simulink model "Normal_Multiplier"  (R2021a)
settings: Solver=FixedStepAuto  StartTime=0.0  StopTime=322.56  FixedStep=0.01  RelTol=1e-3
(part 1 of 3)
settings Model: SimulationMode=rapid-accelerator  Creator=PC  LastModifiedBy=PC
settings DataIOCC: ExternalInput=[u]
settings HardwareCC: ProdHWDeviceType=AMD->x86-64 (Windows64)

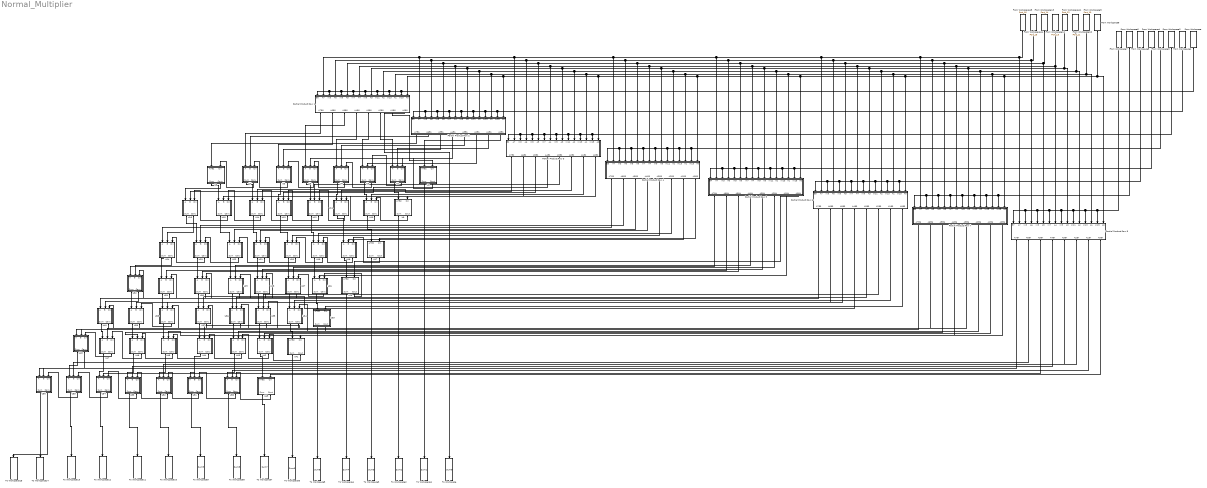
== system Normal_Multiplier ==
  From Workspace : FromWorkspace  VariableName=Port_1
  From Workspace1 : FromWorkspace  VariableName=Port_2
  From Workspace10 : FromWorkspace  VariableName=Port_11
  From Workspace11 : FromWorkspace  VariableName=Port_12
  From Workspace12 : FromWorkspace  VariableName=Port_13
  From Workspace13 : FromWorkspace  VariableName=Port_14
  From Workspace14 : FromWorkspace  VariableName=Port_15
  From Workspace15 : FromWorkspace  VariableName=Port_16
  From Workspace2 : FromWorkspace  VariableName=Port_3
  From Workspace3 : FromWorkspace  VariableName=Port_4
  From Workspace4 : FromWorkspace  VariableName=Port_5
  From Workspace5 : FromWorkspace  VariableName=Port_6
  From Workspace6 : FromWorkspace  VariableName=Port_7
  From Workspace7 : FromWorkspace  VariableName=Port_8
  From Workspace8 : FromWorkspace  VariableName=Port_9
  From Workspace9 : FromWorkspace  VariableName=Port_10
  Partial Product Row 1 : Subsystem
  Partial Product Row 2 : Subsystem
  Partial Product Row 3 : Subsystem
  Partial Product Row 4 : Subsystem
  Partial Product Row 5 : Subsystem
  Partial Product Row 6 : Subsystem
  Partial Product Row 7 : Subsystem
  Partial Product Row 8 : Subsystem
  To Workspace : ToWorkspace  VariableName=Sum0  SampleTime=0.01
      settings: Save2DSignal=2-D array (concatenate along first dimension)
  To Workspace1 : ToWorkspace  VariableName=Sum1  SampleTime=0.01
      settings: Save2DSignal=2-D array (concatenate along first dimension)
  To Workspace10 : ToWorkspace  VariableName=Sum10  SampleTime=0.01
      settings: Save2DSignal=2-D array (concatenate along first dimension)
  To Workspace11 : ToWorkspace  VariableName=Sum11  SampleTime=0.01
      settings: Save2DSignal=2-D array (concatenate along first dimension)
  To Workspace12 : ToWorkspace  VariableName=Sum12  SampleTime=0.01
      settings: Save2DSignal=2-D array (concatenate along first dimension)
  To Workspace13 : ToWorkspace  VariableName=Sum13  SampleTime=0.01
      settings: Save2DSignal=2-D array (concatenate along first dimension)
  To Workspace14 : ToWorkspace  VariableName=Sum14  SampleTime=0.01
      settings: Save2DSignal=2-D array (concatenate along first dimension)
  To Workspace15 : ToWorkspace  VariableName=Sum15  SampleTime=0.01
      settings: Save2DSignal=2-D array (concatenate along first dimension)
  To Workspace2 : ToWorkspace  VariableName=Sum2  SampleTime=0.01
      settings: Save2DSignal=2-D array (concatenate along first dimension)
  To Workspace3 : ToWorkspace  VariableName=Sum3  SampleTime=0.01
      settings: Save2DSignal=2-D array (concatenate along first dimension)
  To Workspace4 : ToWorkspace  VariableName=Sum4  SampleTime=0.01
      settings: Save2DSignal=2-D array (concatenate along first dimension)
  To Workspace5 : ToWorkspace  VariableName=Sum5  SampleTime=0.01
      settings: Save2DSignal=2-D array (concatenate along first dimension)
  To Workspace6 : ToWorkspace  VariableName=Sum6  SampleTime=0.01
      settings: Save2DSignal=2-D array (concatenate along first dimension)
  To Workspace7 : ToWorkspace  VariableName=Sum7  SampleTime=0.01
      settings: Save2DSignal=2-D array (concatenate along first dimension)
  To Workspace8 : ToWorkspace  VariableName=Sum8  SampleTime=0.01
      settings: Save2DSignal=2-D array (concatenate along first dimension)
  To Workspace9 : ToWorkspace  VariableName=Sum9  SampleTime=0.01
      settings: Save2DSignal=2-D array (concatenate along first dimension)
  U1 : Subsystem
  U10 : Subsystem
  U11 : Subsystem
  U12 : Subsystem
  U13 : Subsystem
  U14 : Subsystem
  U15 : Subsystem
  U16 : Subsystem
  U17 : Subsystem
  U18 : Subsystem
  U19 : Subsystem
  U2 : Subsystem
  U20 : Subsystem
  U21 : Subsystem
  U22 : Subsystem
  U23 : Subsystem
  U24 : Subsystem
  U25 : Subsystem
  U26 : Subsystem
  U27 : Subsystem
  U28 : Subsystem
  U29 : Subsystem
  U3 : Subsystem
  U30 : Subsystem
  U31 : Subsystem
  U32 : Subsystem
  U33 : Subsystem
  U34 : Subsystem
  U35 : Subsystem
  U36 : Subsystem
  U37 : Subsystem
  U38 : Subsystem
  U39 : Subsystem
  U4 : Subsystem
  U40 : Subsystem
  U41 : Subsystem
  U42 : Subsystem
  U43 : Subsystem
  U44 : Subsystem
  U45 : Subsystem
  U46 : Subsystem
  U47 : Subsystem
  U48 : Subsystem
  U49 : Subsystem
  U5 : Subsystem
  U50 : Subsystem
  U51 : Subsystem
  U52 : Subsystem
  U53 : Subsystem
  U54 : Subsystem
  U55 : Subsystem
  U56 : Subsystem
  U6 : Subsystem
  U7 : Subsystem
  U8 : Subsystem
  U9 : Subsystem
  wires:
  From Workspace8/1 -> Partial Product Row 8/16(A0), Partial Product Row 7/16(A0), Partial Product Row 6/16(A0), Partial Product Row 4/16(A0), Partial Product Row 3/16(A0), Partial Product Row 1/16(A0), Partial Product Row 2/16(A0), Partial Product Row 5/16(A0)
  From Workspace9/1 -> Partial Product Row 8/14(A1), Partial Product Row 7/14(A1), Partial Product Row 4/14(A1), Partial Product Row 1/14(A1), Partial Product Row 2/14(A1), Partial Product Row 3/14(A1), Partial Product Row 5/14(A1), Partial Product Row 6/14(A1)
  From Workspace10/1 -> Partial Product Row 8/12(A2), Partial Product Row 7/12(A2), Partial Product Row 5/12(A2), Partial Product Row 4/12(A2), Partial Product Row 3/12(A2), Partial Product Row 1/12(A2), Partial Product Row 2/12(A2), Partial Product Row 6/12(A2)
  From Workspace11/1 -> Partial Product Row 8/10(A3), Partial Product Row 6/10(A3), Partial Product Row 4/10(A3), Partial Product Row 3/10(A3), Partial Product Row 1/10(A3), Partial Product Row 2/10(A3), Partial Product Row 5/10(A3), Partial Product Row 7/10(A3)
  From Workspace12/1 -> Partial Product Row 8/8(A4), Partial Product Row 6/8(A4), Partial Product Row 4/8(A4), Partial Product Row 3/8(A4), Partial Product Row 1/8(A4), Partial Product Row 2/8(A4), Partial Product Row 5/8(A4), Partial Product Row 7/8(A4)
  From Workspace13/1 -> Partial Product Row 8/6(A5), Partial Product Row 6/6(A5), Partial Product Row 4/6(A5), Partial Product Row 3/6(A5), Partial Product Row 1/6(A5), Partial Product Row 2/6(A5), Partial Product Row 5/6(A5), Partial Product Row 7/6(A5)
  From Workspace14/1 -> Partial Product Row 8/4(A6), Partial Product Row 7/4(A6), Partial Product Row 6/4(A6), Partial Product Row 5/4(A6), Partial Product Row 4/4(A6), Partial Product Row 3/4(A6), Partial Product Row 1/4(A6), Partial Product Row 2/4(A6)
  From Workspace15/1 -> Partial Product Row 7/2(A7), Partial Product Row 5/2(A7), Partial Product Row 4/2(A7), Partial Product Row 3/2(A7), Partial Product Row 1/2(A7), Partial Product Row 2/2(A7), Partial Product Row 6/2(A7), Partial Product Row 8/2(A7)
  From Workspace/1 -> Partial Product Row 1/3(In3), Partial Product Row 1/1(B0), Partial Product Row 1/5(In5), Partial Product Row 1/7(In7), Partial Product Row 1/9(In9), Partial Product Row 1/11(In11), Partial Product Row 1/13(In13), Partial Product Row 1/15(In15)
  From Workspace1/1 -> Partial Product Row 2/15(In15), Partial Product Row 2/5(In5), Partial Product Row 2/3(In3), Partial Product Row 2/1(B1), Partial Product Row 2/7(In7), Partial Product Row 2/9(In9), Partial Product Row 2/11(In11), Partial Product Row 2/13(In13)
  From Workspace2/1 -> Partial Product Row 3/13(In13), Partial Product Row 3/7(In7), Partial Product Row 3/5(In5), Partial Product Row 3/3(In3), Partial Product Row 3/1(B2), Partial Product Row 3/9(In9), Partial Product Row 3/11(In11), Partial Product Row 3/15(In15)
  From Workspace3/1 -> Partial Product Row 4/15(In15), Partial Product Row 4/13(In13), Partial Product Row 4/11(In11), Partial Product Row 4/9(In9), Partial Product Row 4/7(In7), Partial Product Row 4/5(In5), Partial Product Row 4/1(B3), Partial Product Row 4/3(In3)
  From Workspace4/1 -> Partial Product Row 5/15(In15), Partial Product Row 5/13(In13), Partial Product Row 5/11(In11), Partial Product Row 5/7(In7), Partial Product Row 5/5(In5), Partial Product Row 5/1(B4), Partial Product Row 5/3(In3), Partial Product Row 5/9(In9)
  From Workspace5/1 -> Partial Product Row 6/7(In7), Partial Product Row 6/5(In5), Partial Product Row 6/1(B5), Partial Product Row 6/3(In3), Partial Product Row 6/9(In9), Partial Product Row 6/11(In11), Partial Product Row 6/13(In13), Partial Product Row 6/15(In15)
  From Workspace6/1 -> Partial Product Row 7/13(In13), Partial Product Row 7/7(In7), Partial Product Row 7/5(In5), Partial Product Row 7/1(B6), Partial Product Row 7/3(In3), Partial Product Row 7/9(In9), Partial Product Row 7/11(In11), Partial Product Row 7/15(In15)
  From Workspace7/1 -> Partial Product Row 8/11(In11), Partial Product Row 8/9(In9), Partial Product Row 8/7(In7), Partial Product Row 8/5(In5), Partial Product Row 8/3(In3), Partial Product Row 8/1(B7), Partial Product Row 8/13(In13), Partial Product Row 8/15(In15)
  U17/1(Sum) -> To Workspace3/1
  Partial Product Row 1/8(A0B0) -> To Workspace/1
  U49/2(Cout) -> U50/3(Cin)
  U43/1(Sum) -> U50/1(A)
  U50/2(Carry) -> U51/3(Cin)
  U44/1(Sum) -> U51/1(A)
  U51/2(Carry) -> U52/3(Cin)
  U45/1(Sum) -> U52/1(A)
  U52/2(Carry) -> U53/3(Cin)
  U46/1(Sum) -> U53/1(A)
  U53/2(Carry) -> U54/3(Cin)
  U47/1(Sum) -> U54/1(A)
  U54/2(Carry) -> U55/3(Cin)
  Partial Product Row 1/7(A1B0) -> U1/2(Cin)
  Partial Product Row 2/8(A0B1) -> U1/1(A7B2)
  Partial Product Row 2/7(A1B1) -> U2/2(B)
  Partial Product Row 1/6(A2B0) -> U2/1(A)
  Partial Product Row 1/5(A3B0) -> U3/1(A)
  Partial Product Row 1/4(A4B0) -> U4/1(A)
  Partial Product Row 1/3(A5B0) -> U5/1(A)
  Partial Product Row 1/2(A6B0) -> U6/1(A)
  Partial Product Row 1/1(A7B0) -> U7/1(A)
  U1/2(Cout) -> U2/3(Cin)
  U2/2(Carry) -> U3/3(Cin)
  U3/2(Carry) -> U4/3(Cin)
  U4/2(Carry) -> U5/3(Cin)
  U5/2(Carry) -> U6/3(Cin)
  U6/2(Carry) -> U7/3(Cin)
  U7/2(Carry) -> U8/2(Cin)
  Partial Product Row 2/6(A2B1) -> U3/2(B)
  Partial Product Row 2/5(A3B1) -> U4/2(B)
  Partial Product Row 2/4(A4B1) -> U5/2(B)
  Partial Product Row 2/3(A5B1) -> U6/2(B)
  Partial Product Row 2/2(A6B1) -> U7/2(B)
  Partial Product Row 2/1(A7B1) -> U8/1(A7B2)
  U9/2(Cout) -> U10/3(Cin)
  U10/2(Carry) -> U11/3(Cin)
  U11/2(Carry) -> U12/3(Cin)
  U12/2(Carry) -> U13/3(Cin)
  U13/2(Carry) -> U14/3(Cin)
  U14/2(Carry) -> U15/3(Cin)
  U15/2(Carry) -> U16/3(Cin)
  U8/2(Cout) -> U16/1(A)
  U16/2(Carry) -> U24/2(B)
  U17/2(Cout) -> U18/3(Cin)
  U18/2(Carry) -> U19/3(Cin)
  U19/2(Carry) -> U20/3(Cin)
  U20/2(Carry) -> U21/3(Cin)
  U21/2(Carry) -> U22/3(Cin)
  U22/2(Carry) -> U23/3(Cin)
  U23/2(Carry) -> U24/3(Cin)
  U25/1(Sum) -> To Workspace4/1
  U33/1(Sum) -> To Workspace5/1
  U41/1(Sum) -> To Workspace6/1
  U25/2(Cout) -> U26/3(Cin)
  U26/2(Carry) -> U27/3(Cin)
  U27/2(Carry) -> U28/3(Cin)
  U28/2(Carry) -> U29/3(Cin)
  U29/2(Carry) -> U30/3(Cin)
  U30/2(Carry) -> U31/3(Cin)
  U31/2(Carry) -> U32/3(Cin)
  U24/2(Carry) -> U32/2(B)
  U1/1(Sum) -> To Workspace1/1
  U9/1(Sum) -> To Workspace2/1
  U10/1(Sum) -> U17/1(A7B2)
  U11/1(Sum) -> U18/1(A)
  U12/1(Sum) -> U19/1(A)
  U13/1(Sum) -> U20/1(A)
  U14/1(Sum) -> U21/1(A)
  U15/1(Sum) -> U22/1(A)
  U16/1(Sum) -> U23/1(A)
  U18/1(Sum) -> U25/1(A7B2)
  U19/1(Sum) -> U26/1(A)
  U20/1(Sum) -> U27/1(A)
  U21/1(Sum) -> U28/1(A)
  U22/1(Sum) -> U29/1(A)
  U23/1(Sum) -> U30/1(A)
  U24/1(Sum) -> U31/1(A)
  U26/1(Sum) -> U33/1(A7B2)
  U27/1(Sum) -> U34/1(A)
  U28/1(Sum) -> U35/1(A)
  U29/1(Sum) -> U36/1(A)
  U30/1(Sum) -> U37/1(A)
  U31/1(Sum) -> U38/1(A)
  U32/1(Sum) -> U39/1(A)
  U32/2(Carry) -> U40/2(B)
  U2/1(Sum) -> U9/1(A7B2)
  U3/1(Sum) -> U10/1(A)
  U4/1(Sum) -> U11/1(A)
  U5/1(Sum) -> U12/1(A)
  U6/1(Sum) -> U13/1(A)
  U7/1(Sum) -> U14/1(A)
  U8/1(Sum) -> U15/1(A)
  U34/1(Sum) -> U41/1(A7B2)
  U35/1(Sum) -> U42/1(A)
  U36/1(Sum) -> U43/1(A)
  U37/1(Sum) -> U44/1(A)
  U38/1(Sum) -> U45/1(A)
  U39/1(Sum) -> U46/1(A)
  U40/1(Sum) -> U47/1(A)
  U40/2(Carry) -> U48/2(B)
  U48/2(Carry) -> U56/2(B)
  Partial Product Row 3/8(A0B2) -> U9/2(Cin)
  Partial Product Row 3/7(A1B2) -> U10/2(B)
  Partial Product Row 3/6(A2B2) -> U11/2(B)
  Partial Product Row 3/5(A3B2) -> U12/2(B)
  Partial Product Row 3/4(A4B2) -> U13/2(B)
  Partial Product Row 3/3(A5B2) -> U14/2(B)
  Partial Product Row 3/2(A6B2) -> U15/2(B)
  Partial Product Row 3/1(A7B2) -> U16/2(B)
  Partial Product Row 4/8(A0B3) -> U17/2(Cin)
  Partial Product Row 4/7(A1B3) -> U18/2(B)
  Partial Product Row 4/6(A2B3) -> U19/2(B)
  Partial Product Row 4/5(A3B3) -> U20/2(B)
  Partial Product Row 4/4(A4B3) -> U21/2(B)
  Partial Product Row 4/3(A5B3) -> U22/2(B)
  Partial Product Row 4/2(A6B3) -> U23/2(B)
  Partial Product Row 4/1(A7B3) -> U24/1(A)
  Partial Product Row 5/8(A0B4) -> U25/2(Cin)
  Partial Product Row 5/7(A1B4) -> U26/2(B)
  Partial Product Row 5/6(A2B4) -> U27/2(B)
  Partial Product Row 5/5(A3B4) -> U28/2(B)
  Partial Product Row 5/4(A4B4) -> U29/2(B)
  Partial Product Row 5/3(A5B4) -> U30/2(B)
  Partial Product Row 5/2(A6B4) -> U31/2(B)
  Partial Product Row 5/1(A7B4) -> U32/1(A)
  Partial Product Row 6/8(A0B5) -> U33/2(Cin)
  U33/2(Cout) -> U34/3(Cin)
  U34/2(Carry) -> U35/3(Cin)
  U35/2(Carry) -> U36/3(Cin)
  U36/2(Carry) -> U37/3(Cin)
  U37/2(Carry) -> U38/3(Cin)
  U38/2(Carry) -> U39/3(Cin)
  U39/2(Carry) -> U40/3(Cin)
  Partial Product Row 6/7(A1B5) -> U34/2(B)
  Partial Product Row 6/6(A2B5) -> U35/2(B)
  Partial Product Row 6/5(A3B5) -> U36/2(B)
  Partial Product Row 6/4(A4B5) -> U37/2(B)
  Partial Product Row 6/3(A5B5) -> U38/2(B)
  Partial Product Row 6/2(A6B5) -> U39/2(B)
  Partial Product Row 6/1(A7B5) -> U40/1(A)
  Partial Product Row 7/8(A0B6) -> U41/2(Cin)
  U41/2(Cout) -> U42/3(Cin)
  U42/2(Carry) -> U43/3(Cin)
  U43/2(Carry) -> U44/3(Cin)
  U44/2(Carry) -> U45/3(Cin)
  U45/2(Carry) -> U46/3(Cin)
  U46/2(Carry) -> U47/3(Cin)
  U47/2(Carry) -> U48/3(Cin)
  U48/1(Sum) -> U55/1(A)
  U55/2(Carry) -> U56/3(Cin)
  Partial Product Row 7/7(A1B6) -> U42/2(B)
  Partial Product Row 7/6(A2B6) -> U43/2(B)
  Partial Product Row 7/5(A3B6) -> U44/2(B)
  Partial Product Row 7/4(A4B6) -> U45/2(B)
  Partial Product Row 7/3(A5B6) -> U46/2(B)
  Partial Product Row 7/2(A6B6) -> U47/2(B)
  Partial Product Row 7/1(A7B6) -> U48/1(A)
  U49/1(Sum) -> To Workspace7/1
  U42/1(Sum) -> U49/1(A7B2)
  U50/1(Sum) -> To Workspace8/1
  U51/1(Sum) -> To Workspace9/1
  U52/1(Sum) -> To Workspace10/1
  U53/1(Sum) -> To Workspace11/1
  U54/1(Sum) -> To Workspace12/1
  U55/1(Sum) -> To Workspace13/1
  U56/1(Sum) -> To Workspace14/1
  U56/2(Carry) -> To Workspace15/1
  Partial Product Row 8/8(A0B7) -> U49/2(Cin)
  Partial Product Row 8/7(A1B7) -> U50/2(B)
  Partial Product Row 8/6(A2B7) -> U51/2(B)
  Partial Product Row 8/5(A3B7) -> U52/2(B)
  Partial Product Row 8/4(A4B7) -> U53/2(B)
  Partial Product Row 8/3(A5B7) -> U54/2(B)
  Partial Product Row 8/2(A6B7) -> U55/2(B)
  Partial Product Row 8/1(A7B7) -> U56/1(A)

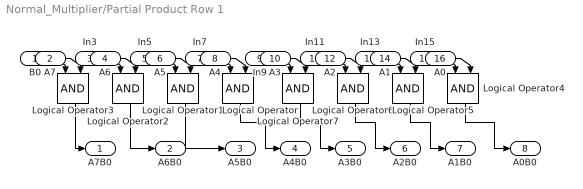
== system Normal_Multiplier/Partial Product Row 1 ==
  B0 : Inport
  A7 : Inport  Port=2
  In3 : Inport  Port=3
  A6 : Inport  Port=4
  In5 : Inport  Port=5
  A5 : Inport  Port=6
  In7 : Inport  Port=7
  A4 : Inport  Port=8
  In9 : Inport  Port=9
  A3 : Inport  Port=10
  In11 : Inport  Port=11
  A2 : Inport  Port=12
  In13 : Inport  Port=13
  A1 : Inport  Port=14
  In15 : Inport  Port=15
  A0 : Inport  Port=16
  Logical Operator{,1..7} (8 alike) : Logic  AllPortsSameDT=off  OutDataTypeStr=boolean
  A7B0 : Outport
  A6B0 : Outport  Port=2
  A5B0 : Outport  Port=3
  A4B0 : Outport  Port=4
  A3B0 : Outport  Port=5
  A2B0 : Outport  Port=6
  A1B0 : Outport  Port=7
  A0B0 : Outport  Port=8
  wires:
  Logical Operator7/1 -> A3B0/1
  Logical Operator4/1 -> A0B0/1
  A4/1 -> Logical Operator/2
  Logical Operator/1 -> A4B0/1
  Logical Operator1/1 -> A5B0/1
  A7/1 -> Logical Operator3/2
  In11/1 -> Logical Operator6/1
  In5/1 -> Logical Operator1/1
  A5/1 -> Logical Operator1/2
  In7/1 -> Logical Operator/1
  A6/1 -> Logical Operator2/2
  B0/1 -> Logical Operator3/1
  A2/1 -> Logical Operator6/2
  Logical Operator3/1 -> A7B0/1
  In3/1 -> Logical Operator2/1
  Logical Operator2/1 -> A6B0/1
  In13/1 -> Logical Operator5/1
  A1/1 -> Logical Operator5/2
  Logical Operator5/1 -> A1B0/1
  Logical Operator6/1 -> A2B0/1
  In9/1 -> Logical Operator7/1
  A3/1 -> Logical Operator7/2
  In15/1 -> Logical Operator4/1
  A0/1 -> Logical Operator4/2

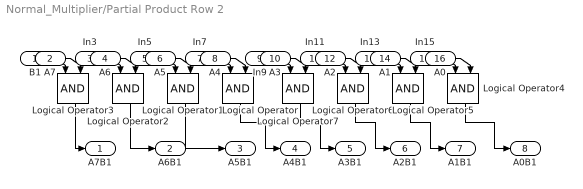
== system Normal_Multiplier/Partial Product Row 2 ==
  B1 : Inport
  A7 : Inport  Port=2
  In3 : Inport  Port=3
  A6 : Inport  Port=4
  In5 : Inport  Port=5
  A5 : Inport  Port=6
  In7 : Inport  Port=7
  A4 : Inport  Port=8
  In9 : Inport  Port=9
  A3 : Inport  Port=10
  In11 : Inport  Port=11
  A2 : Inport  Port=12
  In13 : Inport  Port=13
  A1 : Inport  Port=14
  In15 : Inport  Port=15
  A0 : Inport  Port=16
  Logical Operator{,1..7} (8 alike) : Logic  AllPortsSameDT=off  OutDataTypeStr=boolean
  A7B1 : Outport
  A6B1 : Outport  Port=2
  A5B1 : Outport  Port=3
  A4B1 : Outport  Port=4
  A3B1 : Outport  Port=5
  A2B1 : Outport  Port=6
  A1B1 : Outport  Port=7
  A0B1 : Outport  Port=8
  wires:
  Logical Operator7/1 -> A3B1/1
  Logical Operator4/1 -> A0B1/1
  A4/1 -> Logical Operator/2
  Logical Operator/1 -> A4B1/1
  Logical Operator1/1 -> A5B1/1
  A7/1 -> Logical Operator3/2
  In11/1 -> Logical Operator6/1
  In5/1 -> Logical Operator1/1
  A5/1 -> Logical Operator1/2
  In7/1 -> Logical Operator/1
  A6/1 -> Logical Operator2/2
  B1/1 -> Logical Operator3/1
  A2/1 -> Logical Operator6/2
  Logical Operator3/1 -> A7B1/1
  In3/1 -> Logical Operator2/1
  Logical Operator2/1 -> A6B1/1
  In13/1 -> Logical Operator5/1
  A1/1 -> Logical Operator5/2
  Logical Operator5/1 -> A1B1/1
  Logical Operator6/1 -> A2B1/1
  In9/1 -> Logical Operator7/1
  A3/1 -> Logical Operator7/2
  In15/1 -> Logical Operator4/1
  A0/1 -> Logical Operator4/2

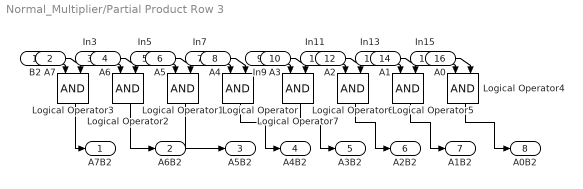
== system Normal_Multiplier/Partial Product Row 3 ==
  B2 : Inport
  A7 : Inport  Port=2
  In3 : Inport  Port=3
  A6 : Inport  Port=4
  In5 : Inport  Port=5
  A5 : Inport  Port=6
  In7 : Inport  Port=7
  A4 : Inport  Port=8
  In9 : Inport  Port=9
  A3 : Inport  Port=10
  In11 : Inport  Port=11
  A2 : Inport  Port=12
  In13 : Inport  Port=13
  A1 : Inport  Port=14
  In15 : Inport  Port=15
  A0 : Inport  Port=16
  Logical Operator{,1..7} (8 alike) : Logic  AllPortsSameDT=off  OutDataTypeStr=boolean
  A7B2 : Outport
  A6B2 : Outport  Port=2
  A5B2 : Outport  Port=3
  A4B2 : Outport  Port=4
  A3B2 : Outport  Port=5
  A2B2 : Outport  Port=6
  A1B2 : Outport  Port=7
  A0B2 : Outport  Port=8
  wires:
  Logical Operator7/1 -> A3B2/1
  Logical Operator4/1 -> A0B2/1
  A4/1 -> Logical Operator/2
  Logical Operator/1 -> A4B2/1
  Logical Operator1/1 -> A5B2/1
  A7/1 -> Logical Operator3/2
  In11/1 -> Logical Operator6/1
  In5/1 -> Logical Operator1/1
  A5/1 -> Logical Operator1/2
  In7/1 -> Logical Operator/1
  A6/1 -> Logical Operator2/2
  B2/1 -> Logical Operator3/1
  A2/1 -> Logical Operator6/2
  Logical Operator3/1 -> A7B2/1
  In3/1 -> Logical Operator2/1
  Logical Operator2/1 -> A6B2/1
  In13/1 -> Logical Operator5/1
  A1/1 -> Logical Operator5/2
  Logical Operator5/1 -> A1B2/1
  Logical Operator6/1 -> A2B2/1
  In9/1 -> Logical Operator7/1
  A3/1 -> Logical Operator7/2
  In15/1 -> Logical Operator4/1
  A0/1 -> Logical Operator4/2

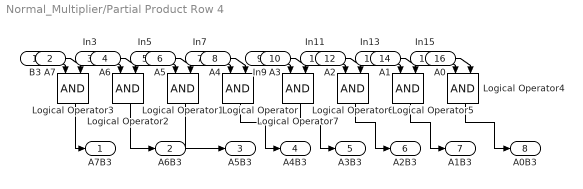
== system Normal_Multiplier/Partial Product Row 4 ==
  B3 : Inport
  A7 : Inport  Port=2
  In3 : Inport  Port=3
  A6 : Inport  Port=4
  In5 : Inport  Port=5
  A5 : Inport  Port=6
  In7 : Inport  Port=7
  A4 : Inport  Port=8
  In9 : Inport  Port=9
  A3 : Inport  Port=10
  In11 : Inport  Port=11
  A2 : Inport  Port=12
  In13 : Inport  Port=13
  A1 : Inport  Port=14
  In15 : Inport  Port=15
  A0 : Inport  Port=16
  Logical Operator{,1..7} (8 alike) : Logic  AllPortsSameDT=off  OutDataTypeStr=boolean
  A7B3 : Outport
  A6B3 : Outport  Port=2
  A5B3 : Outport  Port=3
  A4B3 : Outport  Port=4
  A3B3 : Outport  Port=5
  A2B3 : Outport  Port=6
  A1B3 : Outport  Port=7
  A0B3 : Outport  Port=8
  wires:
  Logical Operator7/1 -> A3B3/1
  Logical Operator4/1 -> A0B3/1
  A4/1 -> Logical Operator/2
  Logical Operator/1 -> A4B3/1
  Logical Operator1/1 -> A5B3/1
  A7/1 -> Logical Operator3/2
  In11/1 -> Logical Operator6/1
  In5/1 -> Logical Operator1/1
  A5/1 -> Logical Operator1/2
  In7/1 -> Logical Operator/1
  A6/1 -> Logical Operator2/2
  B3/1 -> Logical Operator3/1
  A2/1 -> Logical Operator6/2
  Logical Operator3/1 -> A7B3/1
  In3/1 -> Logical Operator2/1
  Logical Operator2/1 -> A6B3/1
  In13/1 -> Logical Operator5/1
  A1/1 -> Logical Operator5/2
  Logical Operator5/1 -> A1B3/1
  Logical Operator6/1 -> A2B3/1
  In9/1 -> Logical Operator7/1
  A3/1 -> Logical Operator7/2
  In15/1 -> Logical Operator4/1
  A0/1 -> Logical Operator4/2

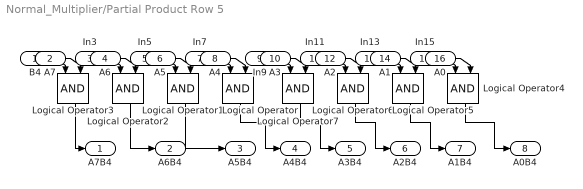
== system Normal_Multiplier/Partial Product Row 5 ==
  B4 : Inport
  A7 : Inport  Port=2
  In3 : Inport  Port=3
  A6 : Inport  Port=4
  In5 : Inport  Port=5
  A5 : Inport  Port=6
  In7 : Inport  Port=7
  A4 : Inport  Port=8
  In9 : Inport  Port=9
  A3 : Inport  Port=10
  In11 : Inport  Port=11
  A2 : Inport  Port=12
  In13 : Inport  Port=13
  A1 : Inport  Port=14
  In15 : Inport  Port=15
  A0 : Inport  Port=16
  Logical Operator{,1..7} (8 alike) : Logic  AllPortsSameDT=off  OutDataTypeStr=boolean
  A7B4 : Outport
  A6B4 : Outport  Port=2
  A5B4 : Outport  Port=3
  A4B4 : Outport  Port=4
  A3B4 : Outport  Port=5
  A2B4 : Outport  Port=6
  A1B4 : Outport  Port=7
  A0B4 : Outport  Port=8
  wires:
  Logical Operator7/1 -> A3B4/1
  Logical Operator4/1 -> A0B4/1
  A4/1 -> Logical Operator/2
  Logical Operator/1 -> A4B4/1
  Logical Operator1/1 -> A5B4/1
  A7/1 -> Logical Operator3/2
  In11/1 -> Logical Operator6/1
  In5/1 -> Logical Operator1/1
  A5/1 -> Logical Operator1/2
  In7/1 -> Logical Operator/1
  A6/1 -> Logical Operator2/2
  B4/1 -> Logical Operator3/1
  A2/1 -> Logical Operator6/2
  Logical Operator3/1 -> A7B4/1
  In3/1 -> Logical Operator2/1
  Logical Operator2/1 -> A6B4/1
  In13/1 -> Logical Operator5/1
  A1/1 -> Logical Operator5/2
  Logical Operator5/1 -> A1B4/1
  Logical Operator6/1 -> A2B4/1
  In9/1 -> Logical Operator7/1
  A3/1 -> Logical Operator7/2
  In15/1 -> Logical Operator4/1
  A0/1 -> Logical Operator4/2

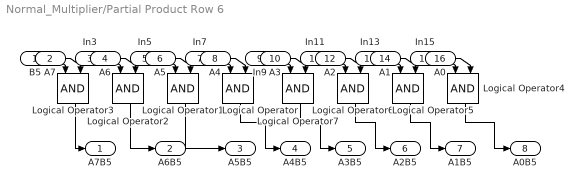
== system Normal_Multiplier/Partial Product Row 6 ==
  B5 : Inport
  A7 : Inport  Port=2
  In3 : Inport  Port=3
  A6 : Inport  Port=4
  In5 : Inport  Port=5
  A5 : Inport  Port=6
  In7 : Inport  Port=7
  A4 : Inport  Port=8
  In9 : Inport  Port=9
  A3 : Inport  Port=10
  In11 : Inport  Port=11
  A2 : Inport  Port=12
  In13 : Inport  Port=13
  A1 : Inport  Port=14
  In15 : Inport  Port=15
  A0 : Inport  Port=16
  Logical Operator{,1..7} (8 alike) : Logic  AllPortsSameDT=off  OutDataTypeStr=boolean
  A7B5 : Outport
  A6B5 : Outport  Port=2
  A5B5 : Outport  Port=3
  A4B5 : Outport  Port=4
  A3B5 : Outport  Port=5
  A2B5 : Outport  Port=6
  A1B5 : Outport  Port=7
  A0B5 : Outport  Port=8
  wires:
  Logical Operator7/1 -> A3B5/1
  Logical Operator4/1 -> A0B5/1
  A4/1 -> Logical Operator/2
  Logical Operator/1 -> A4B5/1
  Logical Operator1/1 -> A5B5/1
  A7/1 -> Logical Operator3/2
  In11/1 -> Logical Operator6/1
  In5/1 -> Logical Operator1/1
  A5/1 -> Logical Operator1/2
  In7/1 -> Logical Operator/1
  A6/1 -> Logical Operator2/2
  B5/1 -> Logical Operator3/1
  A2/1 -> Logical Operator6/2
  Logical Operator3/1 -> A7B5/1
  In3/1 -> Logical Operator2/1
  Logical Operator2/1 -> A6B5/1
  In13/1 -> Logical Operator5/1
  A1/1 -> Logical Operator5/2
  Logical Operator5/1 -> A1B5/1
  Logical Operator6/1 -> A2B5/1
  In9/1 -> Logical Operator7/1
  A3/1 -> Logical Operator7/2
  In15/1 -> Logical Operator4/1
  A0/1 -> Logical Operator4/2

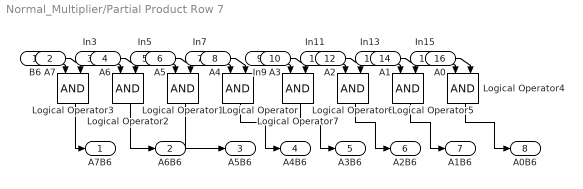
== system Normal_Multiplier/Partial Product Row 7 ==
  B6 : Inport
  A7 : Inport  Port=2
  In3 : Inport  Port=3
  A6 : Inport  Port=4
  In5 : Inport  Port=5
  A5 : Inport  Port=6
  In7 : Inport  Port=7
  A4 : Inport  Port=8
  In9 : Inport  Port=9
  A3 : Inport  Port=10
  In11 : Inport  Port=11
  A2 : Inport  Port=12
  In13 : Inport  Port=13
  A1 : Inport  Port=14
  In15 : Inport  Port=15
  A0 : Inport  Port=16
  Logical Operator{,1..7} (8 alike) : Logic  AllPortsSameDT=off  OutDataTypeStr=boolean
  A7B6 : Outport
  A6B6 : Outport  Port=2
  A5B6 : Outport  Port=3
  A4B6 : Outport  Port=4
  A3B6 : Outport  Port=5
  A2B6 : Outport  Port=6
  A1B6 : Outport  Port=7
  A0B6 : Outport  Port=8
  wires:
  Logical Operator7/1 -> A3B6/1
  Logical Operator4/1 -> A0B6/1
  A4/1 -> Logical Operator/2
  Logical Operator/1 -> A4B6/1
  Logical Operator1/1 -> A5B6/1
  A7/1 -> Logical Operator3/2
  In11/1 -> Logical Operator6/1
  In5/1 -> Logical Operator1/1
  A5/1 -> Logical Operator1/2
  In7/1 -> Logical Operator/1
  A6/1 -> Logical Operator2/2
  B6/1 -> Logical Operator3/1
  A2/1 -> Logical Operator6/2
  Logical Operator3/1 -> A7B6/1
  In3/1 -> Logical Operator2/1
  Logical Operator2/1 -> A6B6/1
  In13/1 -> Logical Operator5/1
  A1/1 -> Logical Operator5/2
  Logical Operator5/1 -> A1B6/1
  Logical Operator6/1 -> A2B6/1
  In9/1 -> Logical Operator7/1
  A3/1 -> Logical Operator7/2
  In15/1 -> Logical Operator4/1
  A0/1 -> Logical Operator4/2

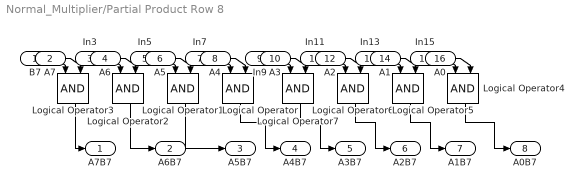
== system Normal_Multiplier/Partial Product Row 8 ==
  B7 : Inport
  A7 : Inport  Port=2
  In3 : Inport  Port=3
  A6 : Inport  Port=4
  In5 : Inport  Port=5
  A5 : Inport  Port=6
  In7 : Inport  Port=7
  A4 : Inport  Port=8
  In9 : Inport  Port=9
  A3 : Inport  Port=10
  In11 : Inport  Port=11
  A2 : Inport  Port=12
  In13 : Inport  Port=13
  A1 : Inport  Port=14
  In15 : Inport  Port=15
  A0 : Inport  Port=16
  Logical Operator{,1..7} (8 alike) : Logic  AllPortsSameDT=off  OutDataTypeStr=boolean
  A7B7 : Outport
  A6B7 : Outport  Port=2
  A5B7 : Outport  Port=3
  A4B7 : Outport  Port=4
  A3B7 : Outport  Port=5
  A2B7 : Outport  Port=6
  A1B7 : Outport  Port=7
  A0B7 : Outport  Port=8
  wires:
  Logical Operator7/1 -> A3B7/1
  Logical Operator4/1 -> A0B7/1
  A4/1 -> Logical Operator/2
  Logical Operator/1 -> A4B7/1
  Logical Operator1/1 -> A5B7/1
  A7/1 -> Logical Operator3/2
  In11/1 -> Logical Operator6/1
  In5/1 -> Logical Operator1/1
  A5/1 -> Logical Operator1/2
  In7/1 -> Logical Operator/1
  A6/1 -> Logical Operator2/2
  B7/1 -> Logical Operator3/1
  A2/1 -> Logical Operator6/2
  Logical Operator3/1 -> A7B7/1
  In3/1 -> Logical Operator2/1
  Logical Operator2/1 -> A6B7/1
  In13/1 -> Logical Operator5/1
  A1/1 -> Logical Operator5/2
  Logical Operator5/1 -> A1B7/1
  Logical Operator6/1 -> A2B7/1
  In9/1 -> Logical Operator7/1
  A3/1 -> Logical Operator7/2
  In15/1 -> Logical Operator4/1
  A0/1 -> Logical Operator4/2

== system Normal_Multiplier/U1 ==
  A7B2 : Inport
  Cin : Inport  Port=2
  Logical Operator : Logic  Operator=XOR  AllPortsSameDT=off  OutDataTypeStr=boolean
  Logical Operator1 : Logic  AllPortsSameDT=off  OutDataTypeStr=boolean
  Sum : Outport
  Cout : Outport  Port=2
  wires:
  A7B2/1 -> Logical Operator1/1, Logical Operator/1
  Cin/1 -> Logical Operator/2, Logical Operator1/2
  Logical Operator/1 -> Sum/1
  Logical Operator1/1 -> Cout/1

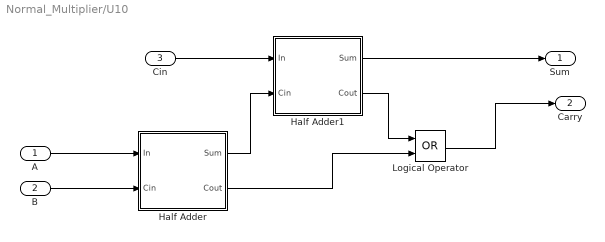
== system Normal_Multiplier/U10 ==
  A : Inport
  B : Inport  Port=2
  Cin : Inport  Port=3
  Half Adder : Subsystem
  Half Adder1 : Subsystem
  Logical Operator : Logic  Operator=OR  AllPortsSameDT=off  OutDataTypeStr=boolean
  Sum : Outport
  Carry : Outport  Port=2
  wires:
  Cin/1 -> Half Adder1/1(In)
  Half Adder1/2(Cout) -> Logical Operator/1
  Half Adder/1(Sum) -> Half Adder1/2(Cin)
  Half Adder1/1(Sum) -> Sum/1
  Half Adder/2(Cout) -> Logical Operator/2
  A/1 -> Half Adder/1(In)
  B/1 -> Half Adder/2(Cin)
  Logical Operator/1 -> Carry/1

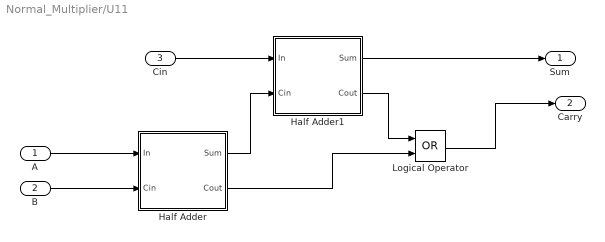
== system Normal_Multiplier/U11 ==
  A : Inport
  B : Inport  Port=2
  Cin : Inport  Port=3
  Half Adder : Subsystem
  Half Adder1 : Subsystem
  Logical Operator : Logic  Operator=OR  AllPortsSameDT=off  OutDataTypeStr=boolean
  Sum : Outport
  Carry : Outport  Port=2
  wires:
  Cin/1 -> Half Adder1/1(In)
  Half Adder1/2(Cout) -> Logical Operator/1
  Half Adder/1(Sum) -> Half Adder1/2(Cin)
  Half Adder1/1(Sum) -> Sum/1
  Half Adder/2(Cout) -> Logical Operator/2
  A/1 -> Half Adder/1(In)
  B/1 -> Half Adder/2(Cin)
  Logical Operator/1 -> Carry/1

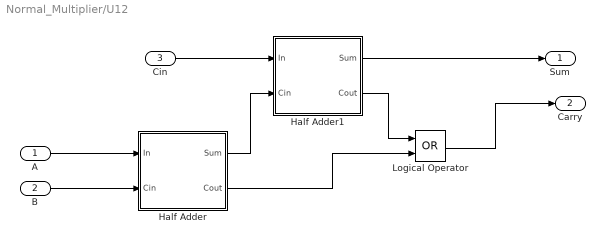
== system Normal_Multiplier/U12 ==
  A : Inport
  B : Inport  Port=2
  Cin : Inport  Port=3
  Half Adder : Subsystem
  Half Adder1 : Subsystem
  Logical Operator : Logic  Operator=OR  AllPortsSameDT=off  OutDataTypeStr=boolean
  Sum : Outport
  Carry : Outport  Port=2
  wires:
  Cin/1 -> Half Adder1/1(In)
  Half Adder1/2(Cout) -> Logical Operator/1
  Half Adder/1(Sum) -> Half Adder1/2(Cin)
  Half Adder1/1(Sum) -> Sum/1
  Half Adder/2(Cout) -> Logical Operator/2
  A/1 -> Half Adder/1(In)
  B/1 -> Half Adder/2(Cin)
  Logical Operator/1 -> Carry/1

== system Normal_Multiplier/U13 ==
  A : Inport
  B : Inport  Port=2
  Cin : Inport  Port=3
  Half Adder : Subsystem
  Half Adder1 : Subsystem
  Logical Operator : Logic  Operator=OR  AllPortsSameDT=off  OutDataTypeStr=boolean
  Sum : Outport
  Carry : Outport  Port=2
  wires:
  Cin/1 -> Half Adder1/1(In)
  Half Adder1/2(Cout) -> Logical Operator/1
  Half Adder/1(Sum) -> Half Adder1/2(Cin)
  Half Adder1/1(Sum) -> Sum/1
  Half Adder/2(Cout) -> Logical Operator/2
  A/1 -> Half Adder/1(In)
  B/1 -> Half Adder/2(Cin)
  Logical Operator/1 -> Carry/1

== system Normal_Multiplier/U14 ==
  A : Inport
  B : Inport  Port=2
  Cin : Inport  Port=3
  Half Adder : Subsystem
  Half Adder1 : Subsystem
  Logical Operator : Logic  Operator=OR  AllPortsSameDT=off  OutDataTypeStr=boolean
  Sum : Outport
  Carry : Outport  Port=2
  wires:
  Cin/1 -> Half Adder1/1(In)
  Half Adder1/2(Cout) -> Logical Operator/1
  Half Adder/1(Sum) -> Half Adder1/2(Cin)
  Half Adder1/1(Sum) -> Sum/1
  Half Adder/2(Cout) -> Logical Operator/2
  A/1 -> Half Adder/1(In)
  B/1 -> Half Adder/2(Cin)
  Logical Operator/1 -> Carry/1

== system Normal_Multiplier/U15 ==
  A : Inport
  B : Inport  Port=2
  Cin : Inport  Port=3
  Half Adder : Subsystem
  Half Adder1 : Subsystem
  Logical Operator : Logic  Operator=OR  AllPortsSameDT=off  OutDataTypeStr=boolean
  Sum : Outport
  Carry : Outport  Port=2
  wires:
  Cin/1 -> Half Adder1/1(In)
  Half Adder1/2(Cout) -> Logical Operator/1
  Half Adder/1(Sum) -> Half Adder1/2(Cin)
  Half Adder1/1(Sum) -> Sum/1
  Half Adder/2(Cout) -> Logical Operator/2
  A/1 -> Half Adder/1(In)
  B/1 -> Half Adder/2(Cin)
  Logical Operator/1 -> Carry/1

== system Normal_Multiplier/U16 ==
  A : Inport
  B : Inport  Port=2
  Cin : Inport  Port=3
  Half Adder : Subsystem
  Half Adder1 : Subsystem
  Logical Operator : Logic  Operator=OR  AllPortsSameDT=off  OutDataTypeStr=boolean
  Sum : Outport
  Carry : Outport  Port=2
  wires:
  Cin/1 -> Half Adder1/1(In)
  Half Adder1/2(Cout) -> Logical Operator/1
  Half Adder/1(Sum) -> Half Adder1/2(Cin)
  Half Adder1/1(Sum) -> Sum/1
  Half Adder/2(Cout) -> Logical Operator/2
  A/1 -> Half Adder/1(In)
  B/1 -> Half Adder/2(Cin)
  Logical Operator/1 -> Carry/1

== system Normal_Multiplier/U17 ==
  A7B2 : Inport
  Cin : Inport  Port=2
  Logical Operator : Logic  Operator=XOR  AllPortsSameDT=off  OutDataTypeStr=boolean
  Logical Operator1 : Logic  AllPortsSameDT=off  OutDataTypeStr=boolean
  Sum : Outport
  Cout : Outport  Port=2
  wires:
  A7B2/1 -> Logical Operator1/1, Logical Operator/1
  Cin/1 -> Logical Operator/2, Logical Operator1/2
  Logical Operator/1 -> Sum/1
  Logical Operator1/1 -> Cout/1

== system Normal_Multiplier/U18 ==
  A : Inport
  B : Inport  Port=2
  Cin : Inport  Port=3
  Half Adder : Subsystem
  Half Adder1 : Subsystem
  Logical Operator : Logic  Operator=OR  AllPortsSameDT=off  OutDataTypeStr=boolean
  Sum : Outport
  Carry : Outport  Port=2
  wires:
  Cin/1 -> Half Adder1/1(In)
  Half Adder1/2(Cout) -> Logical Operator/1
  Half Adder/1(Sum) -> Half Adder1/2(Cin)
  Half Adder1/1(Sum) -> Sum/1
  Half Adder/2(Cout) -> Logical Operator/2
  A/1 -> Half Adder/1(In)
  B/1 -> Half Adder/2(Cin)
  Logical Operator/1 -> Carry/1

== system Normal_Multiplier/U19 ==
  A : Inport
  B : Inport  Port=2
  Cin : Inport  Port=3
  Half Adder : Subsystem
  Half Adder1 : Subsystem
  Logical Operator : Logic  Operator=OR  AllPortsSameDT=off  OutDataTypeStr=boolean
  Sum : Outport
  Carry : Outport  Port=2
  wires:
  Cin/1 -> Half Adder1/1(In)
  Half Adder1/2(Cout) -> Logical Operator/1
  Half Adder/1(Sum) -> Half Adder1/2(Cin)
  Half Adder1/1(Sum) -> Sum/1
  Half Adder/2(Cout) -> Logical Operator/2
  A/1 -> Half Adder/1(In)
  B/1 -> Half Adder/2(Cin)
  Logical Operator/1 -> Carry/1

== system Normal_Multiplier/U2 ==
  A : Inport
  B : Inport  Port=2
  Cin : Inport  Port=3
  Half Adder : Subsystem
  Half Adder1 : Subsystem
  Logical Operator : Logic  Operator=OR  AllPortsSameDT=off  OutDataTypeStr=boolean
  Sum : Outport
  Carry : Outport  Port=2
  wires:
  Cin/1 -> Half Adder1/1(In)
  Half Adder1/2(Cout) -> Logical Operator/1
  Half Adder/1(Sum) -> Half Adder1/2(Cin)
  Half Adder1/1(Sum) -> Sum/1
  Half Adder/2(Cout) -> Logical Operator/2
  A/1 -> Half Adder/1(In)
  B/1 -> Half Adder/2(Cin)
  Logical Operator/1 -> Carry/1

== system Normal_Multiplier/U20 ==
  A : Inport
  B : Inport  Port=2
  Cin : Inport  Port=3
  Half Adder : Subsystem
  Half Adder1 : Subsystem
  Logical Operator : Logic  Operator=OR  AllPortsSameDT=off  OutDataTypeStr=boolean
  Sum : Outport
  Carry : Outport  Port=2
  wires:
  Cin/1 -> Half Adder1/1(In)
  Half Adder1/2(Cout) -> Logical Operator/1
  Half Adder/1(Sum) -> Half Adder1/2(Cin)
  Half Adder1/1(Sum) -> Sum/1
  Half Adder/2(Cout) -> Logical Operator/2
  A/1 -> Half Adder/1(In)
  B/1 -> Half Adder/2(Cin)
  Logical Operator/1 -> Carry/1

== system Normal_Multiplier/U21 ==
  A : Inport
  B : Inport  Port=2
  Cin : Inport  Port=3
  Half Adder : Subsystem
  Half Adder1 : Subsystem
  Logical Operator : Logic  Operator=OR  AllPortsSameDT=off  OutDataTypeStr=boolean
  Sum : Outport
  Carry : Outport  Port=2
  wires:
  Cin/1 -> Half Adder1/1(In)
  Half Adder1/2(Cout) -> Logical Operator/1
  Half Adder/1(Sum) -> Half Adder1/2(Cin)
  Half Adder1/1(Sum) -> Sum/1
  Half Adder/2(Cout) -> Logical Operator/2
  A/1 -> Half Adder/1(In)
  B/1 -> Half Adder/2(Cin)
  Logical Operator/1 -> Carry/1

== system Normal_Multiplier/U22 ==
  A : Inport
  B : Inport  Port=2
  Cin : Inport  Port=3
  Half Adder : Subsystem
  Half Adder1 : Subsystem
  Logical Operator : Logic  Operator=OR  AllPortsSameDT=off  OutDataTypeStr=boolean
  Sum : Outport
  Carry : Outport  Port=2
  wires:
  Cin/1 -> Half Adder1/1(In)
  Half Adder1/2(Cout) -> Logical Operator/1
  Half Adder/1(Sum) -> Half Adder1/2(Cin)
  Half Adder1/1(Sum) -> Sum/1
  Half Adder/2(Cout) -> Logical Operator/2
  A/1 -> Half Adder/1(In)
  B/1 -> Half Adder/2(Cin)
  Logical Operator/1 -> Carry/1

== system Normal_Multiplier/U23 ==
  A : Inport
  B : Inport  Port=2
  Cin : Inport  Port=3
  Half Adder : Subsystem
  Half Adder1 : Subsystem
  Logical Operator : Logic  Operator=OR  AllPortsSameDT=off  OutDataTypeStr=boolean
  Sum : Outport
  Carry : Outport  Port=2
  wires:
  Cin/1 -> Half Adder1/1(In)
  Half Adder1/2(Cout) -> Logical Operator/1
  Half Adder/1(Sum) -> Half Adder1/2(Cin)
  Half Adder1/1(Sum) -> Sum/1
  Half Adder/2(Cout) -> Logical Operator/2
  A/1 -> Half Adder/1(In)
  B/1 -> Half Adder/2(Cin)
  Logical Operator/1 -> Carry/1

== system Normal_Multiplier/U24 ==
  A : Inport
  B : Inport  Port=2
  Cin : Inport  Port=3
  Half Adder : Subsystem
  Half Adder1 : Subsystem
  Logical Operator : Logic  Operator=OR  AllPortsSameDT=off  OutDataTypeStr=boolean
  Sum : Outport
  Carry : Outport  Port=2
  wires:
  Cin/1 -> Half Adder1/1(In)
  Half Adder1/2(Cout) -> Logical Operator/1
  Half Adder/1(Sum) -> Half Adder1/2(Cin)
  Half Adder1/1(Sum) -> Sum/1
  Half Adder/2(Cout) -> Logical Operator/2
  A/1 -> Half Adder/1(In)
  B/1 -> Half Adder/2(Cin)
  Logical Operator/1 -> Carry/1

== system Normal_Multiplier/U25 ==
  A7B2 : Inport
  Cin : Inport  Port=2
  Logical Operator : Logic  Operator=XOR  AllPortsSameDT=off  OutDataTypeStr=boolean
  Logical Operator1 : Logic  AllPortsSameDT=off  OutDataTypeStr=boolean
  Sum : Outport
  Cout : Outport  Port=2
  wires:
  A7B2/1 -> Logical Operator1/1, Logical Operator/1
  Cin/1 -> Logical Operator/2, Logical Operator1/2
  Logical Operator/1 -> Sum/1
  Logical Operator1/1 -> Cout/1

== system Normal_Multiplier/U26 ==
  A : Inport
  B : Inport  Port=2
  Cin : Inport  Port=3
  Half Adder : Subsystem
  Half Adder1 : Subsystem
  Logical Operator : Logic  Operator=OR  AllPortsSameDT=off  OutDataTypeStr=boolean
  Sum : Outport
  Carry : Outport  Port=2
  wires:
  Cin/1 -> Half Adder1/1(In)
  Half Adder1/2(Cout) -> Logical Operator/1
  Half Adder/1(Sum) -> Half Adder1/2(Cin)
  Half Adder1/1(Sum) -> Sum/1
  Half Adder/2(Cout) -> Logical Operator/2
  A/1 -> Half Adder/1(In)
  B/1 -> Half Adder/2(Cin)
  Logical Operator/1 -> Carry/1

== system Normal_Multiplier/U27 ==
  A : Inport
  B : Inport  Port=2
  Cin : Inport  Port=3
  Half Adder : Subsystem
  Half Adder1 : Subsystem
  Logical Operator : Logic  Operator=OR  AllPortsSameDT=off  OutDataTypeStr=boolean
  Sum : Outport
  Carry : Outport  Port=2
  wires:
  Cin/1 -> Half Adder1/1(In)
  Half Adder1/2(Cout) -> Logical Operator/1
  Half Adder/1(Sum) -> Half Adder1/2(Cin)
  Half Adder1/1(Sum) -> Sum/1
  Half Adder/2(Cout) -> Logical Operator/2
  A/1 -> Half Adder/1(In)
  B/1 -> Half Adder/2(Cin)
  Logical Operator/1 -> Carry/1

== system Normal_Multiplier/U28 ==
  A : Inport
  B : Inport  Port=2
  Cin : Inport  Port=3
  Half Adder : Subsystem
  Half Adder1 : Subsystem
  Logical Operator : Logic  Operator=OR  AllPortsSameDT=off  OutDataTypeStr=boolean
  Sum : Outport
  Carry : Outport  Port=2
  wires:
  Cin/1 -> Half Adder1/1(In)
  Half Adder1/2(Cout) -> Logical Operator/1
  Half Adder/1(Sum) -> Half Adder1/2(Cin)
  Half Adder1/1(Sum) -> Sum/1
  Half Adder/2(Cout) -> Logical Operator/2
  A/1 -> Half Adder/1(In)
  B/1 -> Half Adder/2(Cin)
  Logical Operator/1 -> Carry/1

== system Normal_Multiplier/U29 ==
  A : Inport
  B : Inport  Port=2
  Cin : Inport  Port=3
  Half Adder : Subsystem
  Half Adder1 : Subsystem
  Logical Operator : Logic  Operator=OR  AllPortsSameDT=off  OutDataTypeStr=boolean
  Sum : Outport
  Carry : Outport  Port=2
  wires:
  Cin/1 -> Half Adder1/1(In)
  Half Adder1/2(Cout) -> Logical Operator/1
  Half Adder/1(Sum) -> Half Adder1/2(Cin)
  Half Adder1/1(Sum) -> Sum/1
  Half Adder/2(Cout) -> Logical Operator/2
  A/1 -> Half Adder/1(In)
  B/1 -> Half Adder/2(Cin)
  Logical Operator/1 -> Carry/1

== system Normal_Multiplier/U3 ==
  A : Inport
  B : Inport  Port=2
  Cin : Inport  Port=3
  Half Adder : Subsystem
  Half Adder1 : Subsystem
  Logical Operator : Logic  Operator=OR  AllPortsSameDT=off  OutDataTypeStr=boolean
  Sum : Outport
  Carry : Outport  Port=2
  wires:
  Cin/1 -> Half Adder1/1(In)
  Half Adder1/2(Cout) -> Logical Operator/1
  Half Adder/1(Sum) -> Half Adder1/2(Cin)
  Half Adder1/1(Sum) -> Sum/1
  Half Adder/2(Cout) -> Logical Operator/2
  A/1 -> Half Adder/1(In)
  B/1 -> Half Adder/2(Cin)
  Logical Operator/1 -> Carry/1

== system Normal_Multiplier/U30 ==
  A : Inport
  B : Inport  Port=2
  Cin : Inport  Port=3
  Half Adder : Subsystem
  Half Adder1 : Subsystem
  Logical Operator : Logic  Operator=OR  AllPortsSameDT=off  OutDataTypeStr=boolean
  Sum : Outport
  Carry : Outport  Port=2
  wires:
  Cin/1 -> Half Adder1/1(In)
  Half Adder1/2(Cout) -> Logical Operator/1
  Half Adder/1(Sum) -> Half Adder1/2(Cin)
  Half Adder1/1(Sum) -> Sum/1
  Half Adder/2(Cout) -> Logical Operator/2
  A/1 -> Half Adder/1(In)
  B/1 -> Half Adder/2(Cin)
  Logical Operator/1 -> Carry/1

== system Normal_Multiplier/U31 ==
  A : Inport
  B : Inport  Port=2
  Cin : Inport  Port=3
  Half Adder : Subsystem
  Half Adder1 : Subsystem
  Logical Operator : Logic  Operator=OR  AllPortsSameDT=off  OutDataTypeStr=boolean
  Sum : Outport
  Carry : Outport  Port=2
  wires:
  Cin/1 -> Half Adder1/1(In)
  Half Adder1/2(Cout) -> Logical Operator/1
  Half Adder/1(Sum) -> Half Adder1/2(Cin)
  Half Adder1/1(Sum) -> Sum/1
  Half Adder/2(Cout) -> Logical Operator/2
  A/1 -> Half Adder/1(In)
  B/1 -> Half Adder/2(Cin)
  Logical Operator/1 -> Carry/1

== system Normal_Multiplier/U32 ==
  A : Inport
  B : Inport  Port=2
  Cin : Inport  Port=3
  Half Adder : Subsystem
  Half Adder1 : Subsystem
  Logical Operator : Logic  Operator=OR  AllPortsSameDT=off  OutDataTypeStr=boolean
  Sum : Outport
  Carry : Outport  Port=2
  wires:
  Cin/1 -> Half Adder1/1(In)
  Half Adder1/2(Cout) -> Logical Operator/1
  Half Adder/1(Sum) -> Half Adder1/2(Cin)
  Half Adder1/1(Sum) -> Sum/1
  Half Adder/2(Cout) -> Logical Operator/2
  A/1 -> Half Adder/1(In)
  B/1 -> Half Adder/2(Cin)
  Logical Operator/1 -> Carry/1

== system Normal_Multiplier/U33 ==
  A7B2 : Inport
  Cin : Inport  Port=2
  Logical Operator : Logic  Operator=XOR  AllPortsSameDT=off  OutDataTypeStr=boolean
  Logical Operator1 : Logic  AllPortsSameDT=off  OutDataTypeStr=boolean
  Sum : Outport
  Cout : Outport  Port=2
  wires:
  A7B2/1 -> Logical Operator1/1, Logical Operator/1
  Cin/1 -> Logical Operator/2, Logical Operator1/2
  Logical Operator/1 -> Sum/1
  Logical Operator1/1 -> Cout/1

== system Normal_Multiplier/U34 ==
  A : Inport
  B : Inport  Port=2
  Cin : Inport  Port=3
  Half Adder : Subsystem
  Half Adder1 : Subsystem
  Logical Operator : Logic  Operator=OR  AllPortsSameDT=off  OutDataTypeStr=boolean
  Sum : Outport
  Carry : Outport  Port=2
  wires:
  Cin/1 -> Half Adder1/1(In)
  Half Adder1/2(Cout) -> Logical Operator/1
  Half Adder/1(Sum) -> Half Adder1/2(Cin)
  Half Adder1/1(Sum) -> Sum/1
  Half Adder/2(Cout) -> Logical Operator/2
  A/1 -> Half Adder/1(In)
  B/1 -> Half Adder/2(Cin)
  Logical Operator/1 -> Carry/1

== system Normal_Multiplier/U35 ==
  A : Inport
  B : Inport  Port=2
  Cin : Inport  Port=3
  Half Adder : Subsystem
  Half Adder1 : Subsystem
  Logical Operator : Logic  Operator=OR  AllPortsSameDT=off  OutDataTypeStr=boolean
  Sum : Outport
  Carry : Outport  Port=2
  wires:
  Cin/1 -> Half Adder1/1(In)
  Half Adder1/2(Cout) -> Logical Operator/1
  Half Adder/1(Sum) -> Half Adder1/2(Cin)
  Half Adder1/1(Sum) -> Sum/1
  Half Adder/2(Cout) -> Logical Operator/2
  A/1 -> Half Adder/1(In)
  B/1 -> Half Adder/2(Cin)
  Logical Operator/1 -> Carry/1

== system Normal_Multiplier/U36 ==
  A : Inport
  B : Inport  Port=2
  Cin : Inport  Port=3
  Half Adder : Subsystem
  Half Adder1 : Subsystem
  Logical Operator : Logic  Operator=OR  AllPortsSameDT=off  OutDataTypeStr=boolean
  Sum : Outport
  Carry : Outport  Port=2
  wires:
  Cin/1 -> Half Adder1/1(In)
  Half Adder1/2(Cout) -> Logical Operator/1
  Half Adder/1(Sum) -> Half Adder1/2(Cin)
  Half Adder1/1(Sum) -> Sum/1
  Half Adder/2(Cout) -> Logical Operator/2
  A/1 -> Half Adder/1(In)
  B/1 -> Half Adder/2(Cin)
  Logical Operator/1 -> Carry/1

== system Normal_Multiplier/U37 ==
  A : Inport
  B : Inport  Port=2
  Cin : Inport  Port=3
  Half Adder : Subsystem
  Half Adder1 : Subsystem
  Logical Operator : Logic  Operator=OR  AllPortsSameDT=off  OutDataTypeStr=boolean
  Sum : Outport
  Carry : Outport  Port=2
  wires:
  Cin/1 -> Half Adder1/1(In)
  Half Adder1/2(Cout) -> Logical Operator/1
  Half Adder/1(Sum) -> Half Adder1/2(Cin)
  Half Adder1/1(Sum) -> Sum/1
  Half Adder/2(Cout) -> Logical Operator/2
  A/1 -> Half Adder/1(In)
  B/1 -> Half Adder/2(Cin)
  Logical Operator/1 -> Carry/1

== system Normal_Multiplier/U38 ==
  A : Inport
  B : Inport  Port=2
  Cin : Inport  Port=3
  Half Adder : Subsystem
  Half Adder1 : Subsystem
  Logical Operator : Logic  Operator=OR  AllPortsSameDT=off  OutDataTypeStr=boolean
  Sum : Outport
  Carry : Outport  Port=2
  wires:
  Cin/1 -> Half Adder1/1(In)
  Half Adder1/2(Cout) -> Logical Operator/1
  Half Adder/1(Sum) -> Half Adder1/2(Cin)
  Half Adder1/1(Sum) -> Sum/1
  Half Adder/2(Cout) -> Logical Operator/2
  A/1 -> Half Adder/1(In)
  B/1 -> Half Adder/2(Cin)
  Logical Operator/1 -> Carry/1

== system Normal_Multiplier/U39 ==
  A : Inport
  B : Inport  Port=2
  Cin : Inport  Port=3
  Half Adder : Subsystem
  Half Adder1 : Subsystem
  Logical Operator : Logic  Operator=OR  AllPortsSameDT=off  OutDataTypeStr=boolean
  Sum : Outport
  Carry : Outport  Port=2
  wires:
  Cin/1 -> Half Adder1/1(In)
  Half Adder1/2(Cout) -> Logical Operator/1
  Half Adder/1(Sum) -> Half Adder1/2(Cin)
  Half Adder1/1(Sum) -> Sum/1
  Half Adder/2(Cout) -> Logical Operator/2
  A/1 -> Half Adder/1(In)
  B/1 -> Half Adder/2(Cin)
  Logical Operator/1 -> Carry/1

== system Normal_Multiplier/U4 ==
  A : Inport
  B : Inport  Port=2
  Cin : Inport  Port=3
  Half Adder : Subsystem
  Half Adder1 : Subsystem
  Logical Operator : Logic  Operator=OR  AllPortsSameDT=off  OutDataTypeStr=boolean
  Sum : Outport
  Carry : Outport  Port=2
  wires:
  Cin/1 -> Half Adder1/1(In)
  Half Adder1/2(Cout) -> Logical Operator/1
  Half Adder/1(Sum) -> Half Adder1/2(Cin)
  Half Adder1/1(Sum) -> Sum/1
  Half Adder/2(Cout) -> Logical Operator/2
  A/1 -> Half Adder/1(In)
  B/1 -> Half Adder/2(Cin)
  Logical Operator/1 -> Carry/1

== system Normal_Multiplier/U40 ==
  A : Inport
  B : Inport  Port=2
  Cin : Inport  Port=3
  Half Adder : Subsystem
  Half Adder1 : Subsystem
  Logical Operator : Logic  Operator=OR  AllPortsSameDT=off  OutDataTypeStr=boolean
  Sum : Outport
  Carry : Outport  Port=2
  wires:
  Cin/1 -> Half Adder1/1(In)
  Half Adder1/2(Cout) -> Logical Operator/1
  Half Adder/1(Sum) -> Half Adder1/2(Cin)
  Half Adder1/1(Sum) -> Sum/1
  Half Adder/2(Cout) -> Logical Operator/2
  A/1 -> Half Adder/1(In)
  B/1 -> Half Adder/2(Cin)
  Logical Operator/1 -> Carry/1

== system Normal_Multiplier/U41 ==
  A7B2 : Inport
  Cin : Inport  Port=2
  Logical Operator : Logic  Operator=XOR  AllPortsSameDT=off  OutDataTypeStr=boolean
  Logical Operator1 : Logic  AllPortsSameDT=off  OutDataTypeStr=boolean
  Sum : Outport
  Cout : Outport  Port=2
  wires:
  A7B2/1 -> Logical Operator1/1, Logical Operator/1
  Cin/1 -> Logical Operator/2, Logical Operator1/2
  Logical Operator/1 -> Sum/1
  Logical Operator1/1 -> Cout/1

== system Normal_Multiplier/U42 ==
  A : Inport
  B : Inport  Port=2
  Cin : Inport  Port=3
  Half Adder : Subsystem
  Half Adder1 : Subsystem
  Logical Operator : Logic  Operator=OR  AllPortsSameDT=off  OutDataTypeStr=boolean
  Sum : Outport
  Carry : Outport  Port=2
  wires:
  Cin/1 -> Half Adder1/1(In)
  Half Adder1/2(Cout) -> Logical Operator/1
  Half Adder/1(Sum) -> Half Adder1/2(Cin)
  Half Adder1/1(Sum) -> Sum/1
  Half Adder/2(Cout) -> Logical Operator/2
  A/1 -> Half Adder/1(In)
  B/1 -> Half Adder/2(Cin)
  Logical Operator/1 -> Carry/1

== system Normal_Multiplier/U43 ==
  A : Inport
  B : Inport  Port=2
  Cin : Inport  Port=3
  Half Adder : Subsystem
  Half Adder1 : Subsystem
  Logical Operator : Logic  Operator=OR  AllPortsSameDT=off  OutDataTypeStr=boolean
  Sum : Outport
  Carry : Outport  Port=2
  wires:
  Cin/1 -> Half Adder1/1(In)
  Half Adder1/2(Cout) -> Logical Operator/1
  Half Adder/1(Sum) -> Half Adder1/2(Cin)
  Half Adder1/1(Sum) -> Sum/1
  Half Adder/2(Cout) -> Logical Operator/2
  A/1 -> Half Adder/1(In)
  B/1 -> Half Adder/2(Cin)
  Logical Operator/1 -> Carry/1

== system Normal_Multiplier/U44 ==
  A : Inport
  B : Inport  Port=2
  Cin : Inport  Port=3
  Half Adder : Subsystem
  Half Adder1 : Subsystem
  Logical Operator : Logic  Operator=OR  AllPortsSameDT=off  OutDataTypeStr=boolean
  Sum : Outport
  Carry : Outport  Port=2
  wires:
  Cin/1 -> Half Adder1/1(In)
  Half Adder1/2(Cout) -> Logical Operator/1
  Half Adder/1(Sum) -> Half Adder1/2(Cin)
  Half Adder1/1(Sum) -> Sum/1
  Half Adder/2(Cout) -> Logical Operator/2
  A/1 -> Half Adder/1(In)
  B/1 -> Half Adder/2(Cin)
  Logical Operator/1 -> Carry/1

== system Normal_Multiplier/U45 ==
  A : Inport
  B : Inport  Port=2
  Cin : Inport  Port=3
  Half Adder : Subsystem
  Half Adder1 : Subsystem
  Logical Operator : Logic  Operator=OR  AllPortsSameDT=off  OutDataTypeStr=boolean
  Sum : Outport
  Carry : Outport  Port=2
  wires:
  Cin/1 -> Half Adder1/1(In)
  Half Adder1/2(Cout) -> Logical Operator/1
  Half Adder/1(Sum) -> Half Adder1/2(Cin)
  Half Adder1/1(Sum) -> Sum/1
  Half Adder/2(Cout) -> Logical Operator/2
  A/1 -> Half Adder/1(In)
  B/1 -> Half Adder/2(Cin)
  Logical Operator/1 -> Carry/1

== system Normal_Multiplier/U46 ==
  A : Inport
  B : Inport  Port=2
  Cin : Inport  Port=3
  Half Adder : Subsystem
  Half Adder1 : Subsystem
  Logical Operator : Logic  Operator=OR  AllPortsSameDT=off  OutDataTypeStr=boolean
  Sum : Outport
  Carry : Outport  Port=2
  wires:
  Cin/1 -> Half Adder1/1(In)
  Half Adder1/2(Cout) -> Logical Operator/1
  Half Adder/1(Sum) -> Half Adder1/2(Cin)
  Half Adder1/1(Sum) -> Sum/1
  Half Adder/2(Cout) -> Logical Operator/2
  A/1 -> Half Adder/1(In)
  B/1 -> Half Adder/2(Cin)
  Logical Operator/1 -> Carry/1

== system Normal_Multiplier/U47 ==
  A : Inport
  B : Inport  Port=2
  Cin : Inport  Port=3
  Half Adder : Subsystem
  Half Adder1 : Subsystem
  Logical Operator : Logic  Operator=OR  AllPortsSameDT=off  OutDataTypeStr=boolean
  Sum : Outport
  Carry : Outport  Port=2
  wires:
  Cin/1 -> Half Adder1/1(In)
  Half Adder1/2(Cout) -> Logical Operator/1
  Half Adder/1(Sum) -> Half Adder1/2(Cin)
  Half Adder1/1(Sum) -> Sum/1
  Half Adder/2(Cout) -> Logical Operator/2
  A/1 -> Half Adder/1(In)
  B/1 -> Half Adder/2(Cin)
  Logical Operator/1 -> Carry/1

== system Normal_Multiplier/U48 ==
  A : Inport
  B : Inport  Port=2
  Cin : Inport  Port=3
  Half Adder : Subsystem
  Half Adder1 : Subsystem
  Logical Operator : Logic  Operator=OR  AllPortsSameDT=off  OutDataTypeStr=boolean
  Sum : Outport
  Carry : Outport  Port=2
  wires:
  Cin/1 -> Half Adder1/1(In)
  Half Adder1/2(Cout) -> Logical Operator/1
  Half Adder/1(Sum) -> Half Adder1/2(Cin)
  Half Adder1/1(Sum) -> Sum/1
  Half Adder/2(Cout) -> Logical Operator/2
  A/1 -> Half Adder/1(In)
  B/1 -> Half Adder/2(Cin)
  Logical Operator/1 -> Carry/1
